simulink model "Model_vertical"  (R2017b)
settings: Solver=ode4  StartTime=0.0  StopTime=10.0  FixedStep=1e-3  RelTol=1e-3  EnableMultiTasking=on
values from neighbouring files (symbols this model uses):
  a = moment(pwm==0)    [Helicopter_main.m]    (also in Helicopter_main_test.m = moment(pwm==0)/-sin(-0.5223); Lin_simulink.mat = -0.153036; Lin_simulink_test.mat = -0.153036; parametry.m = 0)
  alpha_0 = -28.13    [Helicopter_main.m]    (also in Helicopter_main_test.m = parameters(3); Lin_simulink.mat = -0.522258237308; Lin_simulink_test.mat = -0.52225830565)
  f_v = 0    [Helicopter_main.m]    (also in Helicopter_main_test.m = parameters(2); parametry.m)
  I_v = lsqnonlin(cel, I_v, 0,[],options)    [Helicopter_main.m]    (also in Helicopter_main_test.m; parametry.m = 0)
  J_v = 0    [Helicopter_main.m]    (also in Helicopter_main_test.m = parameters(1); parametry.m)
  lin_alpha_v = pi/18    (= 0.174532925199)    [Helicopter_main_test.m]
  lin_velocity_v = 0    [Helicopter_main_test.m]
  lin_w_v = real(lin_w_v(lin_w_v>-330 & lin_w_v<300 & imag(lin_w_v)==0))    [Helicopter_main_test.m]
  wsp_M_V = polyfit(v/60, moment, 5)    [Helicopter_main.m]    (also in Helicopter_main_test.m = polyfit(v, moment, 5); Lin_simulink.mat = [-2.46242484187e-10 4.61213078344e-09 2.0169387865e-06 1.989; Lin_simulink_test.mat = [-2.51456949125e-14 2.95925329869e-12 8.13117134031e-09 5.04)
  wsp_U_V = polyfit(pred,PWM,5)    [Helicopter_main.m]    (also in Helicopter_main_test.m; Lin_simulink.mat = [-7.28749420126e-10 2.12446681505e-08 6.5068856079e-06 -2.60; Lin_simulink_test.mat = [-7.44181518745e-14 1.363108664e-11 2.62321306545e-08 -6.605)
settings Model: Creator=Student  LastModifiedBy=Marcin
settings DataIOCC: LimitDataPoints=on  SaveFormat=Array
settings OptimizationCC: LifeSpan=inf
settings DebuggingCC: SFUnexpectedBacktrackingDiag=warning  SFNoUnconditionalDefaultTransitionDiag=warning  SFExecutionAtInitializationDiag=none
settings HardwareCC: ProdBitPerPointer=32  ProdBitPerSizeT=32  ProdBitPerPtrDiffT=32  ProdLargestAtomicFloat=None  ProdIntDivRoundTo=Undefined  ProdEndianess=Unspecified  ProdWordSize=32  ProdHWDeviceType=32-bit Generic
settings ModelReferenceCC: PropagateSignalLabelsOutOfModel=off
settings CodeAppCC: StateflowObjectComments=on
settings GRTTargetCC: TargetLangStandard=C89/C90 (ANSI)  GeneratePreprocessorConditionals=Disable all
settings ConfigComp: CovMetricSettings=dw  CovHtmlReporting=on  CovSaveCumulativeToWorkspaceVar=on  CovSaveSingleToWorkspaceVar=on  CovExternalEMLEnable=off

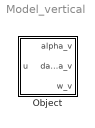
== system Model_vertical ==
  Object : Subsystem

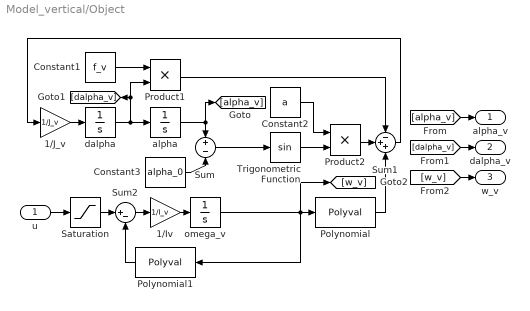
== system Model_vertical/Object ==
  u : Inport
  1/Iv : Gain  Gain=1/I_v
  1/J_v : Gain  Gain=1/J_v
  Constant1 : Constant  Value=f_v
  Constant2 : Constant  Value=a
  Constant3 : Constant  Value=alpha_0
  Polynomial : Polyval  Coefs=wsp_M_V
  Polynomial1 : Polyval  Coefs=wsp_U_V
  Product1 : Product
  Product2 : Product
  Saturation : Saturate  UpperLimit=1  LowerLimit=-1
  Sum : Sum  Inputs=+|-
  Sum1 : Sum  Inputs=-++
  Sum2 : Sum  Inputs=|+-
  Trigonometric Function : Trigonometry
  alpha : Integrator  InitialCondition=lin_alpha_v+0.1
  dalpha : Integrator  InitialCondition=lin_velocity_v
  omega_v : Integrator  InitialCondition=lin_w_v
  alpha_v : Outport
  dalpha_v : Outport  Port=2
  w_v : Outport  Port=3
  wires:
  dalpha/1 -> [dalpha_v], Product1/2, alpha/1
  Trigonometric Function/1 -> Product2/2
  Polynomial1/1 -> Sum2/2
  Sum/1 -> Trigonometric Function/1
  omega_v/1 -> [w_v], Polynomial1/1, Polynomial/1
  Constant2/1 -> Product2/1
  1/J_v/1 -> dalpha/1
  1/Iv/1 -> omega_v/1
  alpha/1 -> [alpha_v], Sum/1
  Sum2/1 -> 1/Iv/1
  Polynomial/1 -> Sum1/3
  Constant3/1 -> Sum/2
  Product2/1 -> Sum1/2
  Constant1/1 -> Product1/1
  Product1/1 -> Sum1/1
  Sum1/1 -> 1/J_v/1
  Saturation/1 -> Sum2/1
  u/1 -> Saturation/1
  [alpha_v] -> alpha_v/1
  [dalpha_v] -> dalpha_v/1
  [w_v] -> w_v/1
